simulink model "SecondOrderCriticallyDampedSystem"  (R2023b)
settings: Solver=VariableStepAuto  StartTime=0.0  StopTime=20  RelTol=1e-3
values from neighbouring files (symbols this model uses):
  G3_den = [B C D]    [SecondOrderOverdampedSystem_SecondOrderCriticallyDampedSystem.m]
  G3_num = [A]    [SecondOrderOverdampedSystem_SecondOrderCriticallyDampedSystem.m]
settings Model: Creator=ASUS Vivobook  LastModifiedBy=ASUS Vivobook

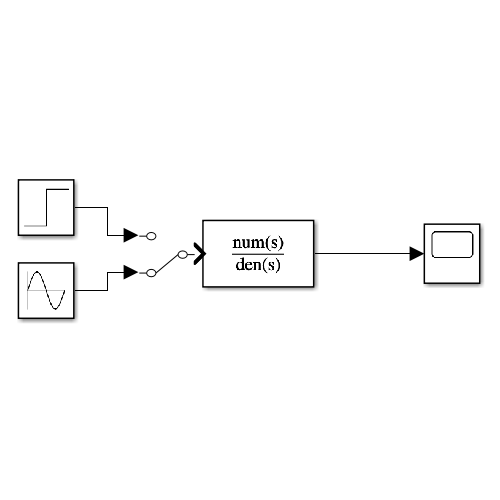
[thumbnail: Simulink's stored preview of the top-level diagram]
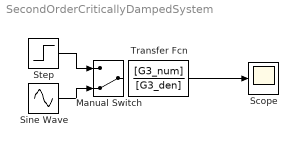
== system SecondOrderCriticallyDampedSystem ==
  Manual Switch : ManualSwitch  CurrentSetting=0
  Scope : Scope
  Sine Wave : Sin  SampleTime=0
  Step : Step  Time=0  SampleTime=0
  Transfer Fcn : TransferFcn  Numerator=[G3_num]  Denominator=[G3_den]
  wires:
  Transfer Fcn/1 -> Scope/1
  Step/1 -> Manual Switch/1
  Sine Wave/1 -> Manual Switch/2
